simulink model "COSTEP"  (R2024b)
settings: Solver=FixedStepAuto  StartTime=0.0  StopTime=25  FixedStep=1/3600  RelTol=1e-3
model workspace (MAT data in the model file):
  AD : Simulink.Parameter (value not decoded)
  AG : Simulink.Parameter (value not decoded)
  AH : Simulink.Parameter (value not decoded)
  AV : Simulink.Parameter (value not decoded)
  AVP : Simulink.Parameter (value not decoded)
  BCHL : Simulink.Parameter (value not decoded)
  BCHV : Simulink.Parameter (value not decoded)
  BD : Simulink.Parameter (value not decoded)
  BDIST : Simulink.Parameter (value not decoded)
  BG : Simulink.Parameter (value not decoded)
  BH : Simulink.Parameter (value not decoded)
  BVP : Simulink.Parameter (value not decoded)
  CD : Simulink.Parameter (value not decoded)
  CDIST : Simulink.Parameter (value not decoded)
  CG : Simulink.Parameter (value not decoded)
  CH : Simulink.Parameter (value not decoded)
  CVP : Simulink.Parameter (value not decoded)
  DDIST : Simulink.Parameter (value not decoded)
  DIST_CONST : Simulink.Parameter (value not decoded)
  ISV : Simulink.Parameter (value not decoded)
  TLAST : Simulink.Parameter (value not decoded)
  TNEXT : Simulink.Parameter (value not decoded)
  XMW : Simulink.Parameter (value not decoded)
  XNS : Simulink.Parameter (value not decoded)
  XNS2 : Simulink.Parameter (value not decoded)
  XNS3 : Simulink.Parameter (value not decoded)
  XNSADD : Simulink.Parameter (value not decoded)
  XNSE : Simulink.Parameter (value not decoded)
symbols that are objects in the model workspace (value not decoded): AD, AG, AH, AV, AVP, BD, BG, BH, BVP, CD, CG, CH, CVP, XMW, XNS, XNS2, XNS3, XNSE
undefined symbols (not defined in the file or in its folder): magnitude, msgbox, SETPT, XMEAS, XMV
libraries: mylib x381, dspindex x31
(part 4 of 12)

== system COSTEP/Stripper/PTC Pressure of Liquid zone in stripper mmHg ==
  XLC : Inport
  TCC : Inport  Port=2
  Bus Creator1 : BusCreator  Inputs=8
  Demux : Demux  Outputs=8
  PPR(I) : Product
  PTR Total Pressure of Reactor mmHg : Sum  Inputs=+
  VPR Vapour Pressure mmHg : Subsystem
  PTC : Outport  PortDimensions=1  VectorParamsAs1DForOutWhenUnconnected=off
  wires:
  Demux/1 -> Bus Creator1/1  "PPR(1)"
  Demux/2 -> Bus Creator1/2  "PPR(2)"
  Demux/7 -> Bus Creator1/7  "PPR(7)"
  TCC/1 -> VPR Vapour Pressure mmHg/1(TCR)
  Demux/8 -> Bus Creator1/8  "PPR(8)"
  PPR(I)/1 -> Demux/1
  VPR Vapour Pressure mmHg/1(VPR) -> PPR(I)/2
  PTR Total Pressure of Reactor mmHg/1 -> PTC/1
  XLC/1 -> PPR(I)/1
  Bus Creator1/1 -> PTR Total Pressure of Reactor mmHg/1
  Demux/6 -> Bus Creator1/6  "PPR(6)"
  Demux/4 -> Bus Creator1/4  "PPR(4)"
  Demux/5 -> Bus Creator1/5  "PPR(5)"
  Demux/3 -> Bus Creator1/3  "PPR(3)"

== system COSTEP/Stripper/Position of Valve 8 % ==
  Bus Selector : BusSelector  OutputSignals=XMV(8)
  Bus Selector1 : BusSelector  OutputSignals=IDV(19)
  Constant : Constant  Value=46
  Control valve : mylib/Control valve  SystemSampleTime=-1  VariantActivationTime=update diagram  AllowFlexibleInterface=on  Latency=0  AutoFrameSizeCalculation=off
  Divide : Product  Inputs=*/
  Initial state variable : mylib/Initial state variable
  Integration : mylib/Integration  SystemSampleTime=-1  VariantActivationTime=update diagram  AllowFlexibleInterface=on  Latency=0  AutoFrameSizeCalculation=off
  Subtract : Sum  Inputs=+-
  VTAU(8) : Constant  Value=5/3600
  "YY(46) " : Outport  PortDimensions=1  VectorParamsAs1DForOutWhenUnconnected=off
  wires:
  Integration/1 -> "YY(46) "/1, Subtract/2  "VPOS(8)"
  Subtract/1 -> Divide/1
  Control valve/1 -> Subtract/1
  VTAU(8)/1 -> Divide/2
  Divide/1 -> Integration/1
  Initial state variable/1 -> Integration/2
  [XMV] -> Bus Selector/1
  Bus Selector/1 -> Control valve/1  "<XMV(8)>"
  [IDV] -> Bus Selector1/1
  Bus Selector1/1 -> Control valve/2  "<IDV(19)>"
  Constant/1 -> Initial state variable/1

== system COSTEP/Stripper/Position of Valve 9 % ==
  Bus Selector : BusSelector  OutputSignals=XMV(9)
  Bus Selector1 : BusSelector  OutputSignals=IDV(19)
  Constant : Constant  Value=47
  Control valve : mylib/Control valve  SystemSampleTime=-1  VariantActivationTime=update diagram  AllowFlexibleInterface=on  Latency=0  AutoFrameSizeCalculation=off
  Divide : Product  Inputs=*/
  Initial state variable : mylib/Initial state variable
  Integration : mylib/Integration  SystemSampleTime=-1  VariantActivationTime=update diagram  AllowFlexibleInterface=on  Latency=0  AutoFrameSizeCalculation=off
  Subtract : Sum  Inputs=+-
  VTAU(9) : Constant  Value=120/3600
  "YY(47) " : Outport  PortDimensions=1  VectorParamsAs1DForOutWhenUnconnected=off
  wires:
  Integration/1 -> "YY(47) "/1, Subtract/2  "VPOS(9)"
  Subtract/1 -> Divide/1
  Control valve/1 -> Subtract/1
  VTAU(9)/1 -> Divide/2
  Divide/1 -> Integration/1
  Initial state variable/1 -> Integration/2
  [XMV] -> Bus Selector/1
  Bus Selector/1 -> Control valve/1  "<XMV(9)>"
  Bus Selector1/1 -> Control valve/2  "<IDV(19)>"
  [IDV] -> Bus Selector1/1
  Constant/1 -> Initial state variable/1

== system COSTEP/Stripper/Split Fractions ==
  Bus Creator1 : BusCreator  Inputs=4
  SFR(1) : Constant  Value=0.99500
  SFR(2) : Constant  Value=0.99100
  SFR(3) : Constant  Value=0.99000
  Split fraction : Subsystem
  SFR : Outport  VectorParamsAs1DForOutWhenUnconnected=off
  wires:
  Bus Creator1/1 -> SFR/1
  SFR(2)/1 -> Bus Creator1/2
  Split fraction/1(SFR) -> Bus Creator1/4
  SFR(1)/1 -> Bus Creator1/1
  SFR(3)/1 -> Bus Creator1/3

== system COSTEP/Stripper/Stream 12 ==
  FCM(I,12) : Inport
  Bus Creator : BusCreator  Inputs=5
  Display : Display
  FTM(12) : Sum  Inputs=+
  Gain : Gain
  HST(12) Molar Enthalpy of Stream 12 MBtu/lb-mol : Subsystem
  ITY : Constant  Value=0
  XST(I,12) : Product  Inputs=*/
  wires:
  FTM(12)/1 -> XST(I,12)/2, Bus Creator/4  "FTM(12)"
  FCM(I,12)/1 -> XST(I,12)/1, Bus Creator/5, FTM(12)/1  "FCM(I;12)"
  XST(I,12)/1 -> Bus Creator/1, HST(12) Molar Enthalpy of Stream 12 MBtu/lb-mol/3(XST(I,I))  "XST(I;12)"
  [TCC] -> Gain/1
  Gain/1 -> Bus Creator/2, HST(12) Molar Enthalpy of Stream 12 MBtu/lb-mol/2(T)  "TST(12)"
  ITY/1 -> HST(12) Molar Enthalpy of Stream 12 MBtu/lb-mol/1(ITY)
  HST(12) Molar Enthalpy of Stream 12 MBtu/lb-mol/1("H ") -> Bus Creator/3  "HST(12)"
  Bus Creator/1 -> Display/1

== system COSTEP/Stripper/Stream 13 ==
  XST(I,13) : Inport  PortDimensions=8
  TST(13) : Inport  Port=2
  VPOS(8) : Inport  Port=3
  PTC : Inport  Port=4
  "   " : Constant  Value=100
  Bus Creator : BusCreator  Inputs=7
  FCM(I,13) Component molar flow of Stream 13 lb-mol/h : Product
  FTM(13) : Product  Inputs=**/
  HST(13) Molar Enthalpy of Stream 13 MBtu/lb-mol : Subsystem
  ITY : Constant  Value=0
  VRNG(8) : Constant  Value=1000
  Properties of Stream 13 : Outport  VectorParamsAs1DForOutWhenUnconnected=off
  wires:
  FTM(13)/1 -> Bus Creator/4, FCM(I,13) Component molar flow of Stream 13 lb-mol/h/2  "FTM(13)"
  ITY/1 -> Bus Creator/6, HST(13) Molar Enthalpy of Stream 13 MBtu/lb-mol/1(ITY)  "Phase"
  XST(I,13)/1 -> Bus Creator/1, FCM(I,13) Component molar flow of Stream 13 lb-mol/h/1, HST(13) Molar Enthalpy of Stream 13 MBtu/lb-mol/3(XST(I,I))  "XST(I;13)"
  HST(13) Molar Enthalpy of Stream 13 MBtu/lb-mol/1("H ") -> Bus Creator/3  "HST(13)"
  TST(13)/1 -> Bus Creator/2, HST(13) Molar Enthalpy of Stream 13 MBtu/lb-mol/2(T)  "TST(13)"
  VPOS(8)/1 -> FTM(13)/1
  FCM(I,13) Component molar flow of Stream 13 lb-mol/h/1 -> Bus Creator/5  "FCM(I;13)"
  VRNG(8)/1 -> FTM(13)/2
  "   "/1 -> FTM(13)/3
  Bus Creator/1 -> Properties of Stream 13/1
  PTC/1 -> Bus Creator/7  "PTC"

== system COSTEP/Stripper/Stream 5 ==
  FCM(I,5) : Inport
  Bus Creator : BusCreator  Inputs=7
  FTM(5) : Sum  Inputs=+
  HST(5) Molar Enthalpy of Stream 5 MBtu/lb-mol : Subsystem
  ITY : Constant
  XST(I,5) : Product  Inputs=*/
  Properties of Stream 5 : Outport  VectorParamsAs1DForOutWhenUnconnected=off
  tag scope: PropertiesStream5=global
  wires:
  FTM(5)/1 -> Bus Creator/4, XST(I,5)/2  "FTM(5)"
  FCM(I,5)/1 -> XST(I,5)/1, Bus Creator/5, FTM(5)/1  "FCM(I;5)"
  XST(I,5)/1 -> Bus Creator/1, HST(5) Molar Enthalpy of Stream 5 MBtu/lb-mol/3(XST(I,5))  "XST(I;5)"
  [TCC] -> Bus Creator/2, HST(5) Molar Enthalpy of Stream 5 MBtu/lb-mol/2(TST(5))  "TST(5)"
  ITY/1 -> Bus Creator/6, HST(5) Molar Enthalpy of Stream 5 MBtu/lb-mol/1(ITY)  "Phase"
  HST(5) Molar Enthalpy of Stream 5 MBtu/lb-mol/1("H ") -> Bus Creator/3  "HST(5)"
  Bus Creator/1 -> [PropertiesStream5], Properties of Stream 5/1
  [PTV] -> Bus Creator/7

== system COSTEP/Stripper/TCC Initial Temperature in Stripper °C  ==
  UTLC : Inport  PortDimensions=1
  ETC : Inport  Port=2  PortDimensions=1
  XLC : Inport  Port=3  PortDimensions=8
  "AG(I) Coefficient A to determine Enthalpy MBtu/lb·°F " : Constant  Value=[3.411e-6;0.3799e-6;0.2491e-6;0.3567e-6;0.3463e-6;0.393e-6;0.17e-6;0.15e-6]
  "AH(I) Coefficient A to determine Enthalpy MBtu/lb·°F " : Constant  Value=[1e-6;1e-6;1e-6;0.96e-6;0.573e-6;0.652e-6;0.515e-6;0.471e-6]
  AV(I) Coefficient AV to determine Enthalpy MBtu/lb : Constant  Value=[1e-6;1e-6;1e-6;86.7e-6;160e-6;160e-6;225e-6;209e-6]
  BG(I) Coefficient B to determine Enthalpy MBtu/lb·°F² : Constant  Value=[7.18e-10;1.08e-9;1.36e-11;8.51e-10;8.96e-10;1.02e-9;0;0]
  BH(I) Coefficient B to determine Enthalpy MBtu/lb·°F² : Constant  Value=[0;0;0;8.7e-9;2.41e-9;2.18e-9;5.65e-10;8.7e-10]
  CG(I) Coefficient C to determine Enthalpy MBtu/lb·°F³ : Constant  Value=[6e-13;-3.98e-13;-3.93e-14;-3.12e-13;-3.27e-13;-3.12e-13;0;0]
  CH(I) Coefficient C to determine Enthalpy MBtu/lb·°F³ : Constant  Value=[0;0;0;4.81e-11;1.82e-11;1.94e-11;3.82e-12;2.62e-12]
  Delay : Delay  DelayLength=1  InitialCondition=0
  ITY : Constant  Value=0
  MATLAB Function : MATLAB Function  TreatAsAtomicUnit=on
  "XMW(I) Molecular weight of components lb/lb-mol " : Constant  Value=[2;25.4;28;32;46;48;62;76]
  TCC : Outport  PortDimensions=1  VectorParamsAs1DForOutWhenUnconnected=off
  wires:
  MATLAB Function/1(TCC) -> Delay/1, TCC/1
  Delay/1 -> MATLAB Function/13("TCC ")
  "AG(I) Coefficient A to determine Enthalpy MBtu/lb·°F "/1 -> MATLAB Function/4(AG)
  AV(I) Coefficient AV to determine Enthalpy MBtu/lb/1 -> MATLAB Function/7(AV)
  ETC/1 -> MATLAB Function/10(ETC)
  CH(I) Coefficient C to determine Enthalpy MBtu/lb·°F³/1 -> MATLAB Function/3(CH)
  UTLC/1 -> MATLAB Function/11(UTLC)
  ITY/1 -> MATLAB Function/12(ITY)
  "XMW(I) Molecular weight of components lb/lb-mol "/1 -> MATLAB Function/8(XMW)
  XLC/1 -> MATLAB Function/9(XLC)
  "AH(I) Coefficient A to determine Enthalpy MBtu/lb·°F "/1 -> MATLAB Function/1(AH)
  CG(I) Coefficient C to determine Enthalpy MBtu/lb·°F³/1 -> MATLAB Function/6(CG)
  BH(I) Coefficient B to determine Enthalpy MBtu/lb·°F²/1 -> MATLAB Function/2(BH)
  BG(I) Coefficient B to determine Enthalpy MBtu/lb·°F²/1 -> MATLAB Function/5(BG)

== system COSTEP/Stripper/Volume of Stripper ==
  UTLC : Inport  PortDimensions=1
  XLC : Inport  Port=2  PortDimensions=8
  "DLC Molar Density of Liquids in Stripper lb-mol/ft³    " : Subsystem
  "VLC Liquid Volume in Stripper ft³ " : Product  Inputs=*/
  tag scope: DLC=global, VLC=global
  wires:
  "DLC Molar Density of Liquids in Stripper lb-mol/ft³    "/1("DLC ") -> [DLC], "VLC Liquid Volume in Stripper ft³ "/2
  XLC/1 -> "DLC Molar Density of Liquids in Stripper lb-mol/ft³    "/1(XLC)
  "VLC Liquid Volume in Stripper ft³ "/1 -> [VLC]
  [TCC] -> "DLC Molar Density of Liquids in Stripper lb-mol/ft³    "/2(TCC)
  UTLC/1 -> "VLC Liquid Volume in Stripper ft³ "/1

== system COSTEP/Valve/FTM(1) Total molar flow of Stream 1 lb-mol//h ==
  VPOS(1) : Inport
  VRNG(1) : Inport  Port=2
  " " : Product  Inputs=**/
  Constant : Constant  Value=100
  FTM(1) : Outport  PortDimensions=1  VectorParamsAs1DForOutWhenUnconnected=off
  wires:
  VRNG(1)/1 -> " "/2
  Constant/1 -> " "/3
  VPOS(1)/1 -> " "/1
  " "/1 -> FTM(1)/1

== system COSTEP/Valve/Position of Valve 1 % ==
  Bus Selector : BusSelector  OutputSignals=XMV(1)
  Constant : Constant  Value=39
  Control valve : mylib/Control valve  SystemSampleTime=-1  VariantActivationTime=update diagram  AllowFlexibleInterface=on  Latency=0  AutoFrameSizeCalculation=off
  Divide : Product  Inputs=*/
  IVST(1) : Constant  Value=0
  Initial state variable : mylib/Initial state variable
  Integration : mylib/Integration  SystemSampleTime=-1  VariantActivationTime=update diagram  AllowFlexibleInterface=on  Latency=0  AutoFrameSizeCalculation=off
  Subtract : Sum  Inputs=+-
  VTAU(1) : Constant  Value=8/3600
  "YY(39) " : Outport  VectorParamsAs1DForOutWhenUnconnected=off
  wires:
  Integration/1 -> "YY(39) "/1, Subtract/2  "VPOS(1)"
  Subtract/1 -> Divide/1
  VTAU(1)/1 -> Divide/2
  Divide/1 -> Integration/1
  Control valve/1 -> Subtract/1
  [XMV] -> Bus Selector/1
  Bus Selector/1 -> Control valve/1  "<XMV(1)>"
  IVST(1)/1 -> Control valve/2
  Constant/1 -> Initial state variable/1
  Initial state variable/1 -> Integration/2

== system COSTEP/Valve 2/FTM(2) Total molar flow of Stream 2 lb-mol//h ==
  VPOS(2) : Inport
  VRNG(2) : Inport  Port=2
  " " : Product  Inputs=**/
  Constant : Constant  Value=100
  FTM(2) : Outport  PortDimensions=1  VectorParamsAs1DForOutWhenUnconnected=off
  wires:
  VRNG(2)/1 -> " "/2
  Constant/1 -> " "/3
  VPOS(2)/1 -> " "/1
  " "/1 -> FTM(2)/1

== system COSTEP/Valve 2/Position of Valve 2 % ==
  Bus Selector : BusSelector  OutputSignals=XMV(2)
  Constant : Constant  Value=40
  Control valve : mylib/Control valve  SystemSampleTime=-1  VariantActivationTime=update diagram  AllowFlexibleInterface=on  Latency=0  AutoFrameSizeCalculation=off
  Divide : Product  Inputs=*/
  IVST(2) : Constant  Value=0
  Initial state variable : mylib/Initial state variable
  Integration : mylib/Integration  SystemSampleTime=-1  VariantActivationTime=update diagram  AllowFlexibleInterface=on  Latency=0  AutoFrameSizeCalculation=off
  Subtract : Sum  Inputs=+-
  VTAU(2) : Constant  Value=8/3600
  "YY(40)  " : Outport  VectorParamsAs1DForOutWhenUnconnected=off
  wires:
  Control valve/1 -> Subtract/1
  Subtract/1 -> Divide/1
  VTAU(2)/1 -> Divide/2
  Divide/1 -> Integration/1
  Integration/1 -> Subtract/2, "YY(40)  "/1  "VPOS(2)"
  Initial state variable/1 -> Integration/2
  [XMV] -> Bus Selector/1
  Bus Selector/1 -> Control valve/1  "<XMV(2)>"
  IVST(2)/1 -> Control valve/2
  Constant/1 -> Initial state variable/1

== system COSTEP/Valve 3/FTM(3) Total molar flow of Stream 3 lb-mol//h ==
  VPOS(3) : Inport
  VRNG(3) : Inport  Port=2
  " " : Product  Inputs=***/
  Bus Selector : BusSelector  OutputSignals=IDV(6)
  Constant : Constant  Value=100
  Constant1 : Constant
  Subtract : Sum  Inputs=+-
  FTM(3) : Outport  PortDimensions=1  VectorParamsAs1DForOutWhenUnconnected=off
  wires:
  VPOS(3)/1 -> " "/1
  " "/1 -> FTM(3)/1
  Constant1/1 -> Subtract/1
  [IDV] -> Bus Selector/1
  Constant/1 -> " "/4
  Subtract/1 -> " "/2
  VRNG(3)/1 -> " "/3
  Bus Selector/1 -> Subtract/2  "<IDV(6)>"

== system COSTEP/Valve 3/Position of Valve 3 % ==
  Bus Selector : BusSelector  OutputSignals=XMV(3)
  Constant : Constant  Value=41
  Control valve : mylib/Control valve  SystemSampleTime=-1  VariantActivationTime=update diagram  AllowFlexibleInterface=on  Latency=0  AutoFrameSizeCalculation=off
  Divide : Product  Inputs=*/
  IVST(3) : Constant  Value=0
  Initial state variable : mylib/Initial state variable
  Integration : mylib/Integration  SystemSampleTime=-1  VariantActivationTime=update diagram  AllowFlexibleInterface=on  Latency=0  AutoFrameSizeCalculation=off
  Subtract : Sum  Inputs=+-
  VTAU(3) : Constant  Value=6/3600
  "YY(41) " : Outport  VectorParamsAs1DForOutWhenUnconnected=off
  wires:
  Control valve/1 -> Subtract/1
  Subtract/1 -> Divide/1
  VTAU(3)/1 -> Divide/2
  Divide/1 -> Integration/1
  Integration/1 -> "YY(41) "/1, Subtract/2  "VPOS(3)"
  Initial state variable/1 -> Integration/2
  [XMV] -> Bus Selector/1
  Bus Selector/1 -> Control valve/1  "<XMV(3)>"
  IVST(3)/1 -> Control valve/2
  Constant/1 -> Initial state variable/1

== system COSTEP/Valve 4/FTM(4) Total molar flow of Stream 4 lb-mol//h ==
  VPOS(4) : Inport
  VRNG(4) : Inport  Port=2
  " " : Product  Inputs=***/
  Add : Sum
  Bus Selector : BusSelector  OutputSignals=IDV(7)
  Constant : Constant
  Constant1 : Constant  Value=0.2
  Constant3 : Constant  Value=100
  Constant4 : Constant  Value=1e-10
  Product1 : Product
  Subtract : Sum  Inputs=+-
  FTM(4) : Outport  PortDimensions=1  VectorParamsAs1DForOutWhenUnconnected=off
  wires:
  Add/1 -> FTM(4)/1
  Constant4/1 -> Add/2
  " "/1 -> Add/1
  VPOS(4)/1 -> " "/1
  Bus Selector/1 -> Product1/1  "<IDV(7)>"
  Product1/1 -> Subtract/2
  Constant1/1 -> Product1/2
  Constant/1 -> Subtract/1
  Constant3/1 -> " "/4
  VRNG(4)/1 -> " "/3
  Subtract/1 -> " "/2
  [IDV] -> Bus Selector/1

== system COSTEP/Valve 4/Position of Valve 4 % ==
  Bus Selector : BusSelector  OutputSignals=XMV(4)
  Constant : Constant  Value=42
  Control valve : mylib/Control valve  SystemSampleTime=-1  VariantActivationTime=update diagram  AllowFlexibleInterface=on  Latency=0  AutoFrameSizeCalculation=off
  Divide : Product  Inputs=*/
  IVST(4) : Constant  Value=0
  Initial state variable : mylib/Initial state variable
  Integration : mylib/Integration  SystemSampleTime=-1  VariantActivationTime=update diagram  AllowFlexibleInterface=on  Latency=0  AutoFrameSizeCalculation=off
  Subtract : Sum  Inputs=+-
  VTAU(4) : Constant  Value=9/3600
  "YY(42) " : Outport  VectorParamsAs1DForOutWhenUnconnected=off
  wires:
  Control valve/1 -> Subtract/1
  Subtract/1 -> Divide/1
  VTAU(4)/1 -> Divide/2
  Divide/1 -> Integration/1
  Integration/1 -> "YY(42) "/1, Subtract/2  "VPOS(4)"
  Initial state variable/1 -> Integration/2
  [XMV] -> Bus Selector/1
  Bus Selector/1 -> Control valve/1  "<XMV(4)>"
  IVST(4)/1 -> Control valve/2
  Constant/1 -> Initial state variable/1

== system COSTEP/Compressor/Subsystem/If Action Subsystem ==
  In1 : Inport
  Action Port : ActionPort  ActionPortLabel=if(u1 < 1)
  Out1 : Outport  VectorParamsAs1DForOutWhenUnconnected=off
  wires:
  In1/1 -> Out1/1

== system COSTEP/Compressor/Subsystem/If Action Subsystem1 ==
  In1 : Inport
  Action Port : ActionPort  ActionPortLabel=elseif(u1>1.3)
  Out1 : Outport  VectorParamsAs1DForOutWhenUnconnected=off
  wires:
  In1/1 -> Out1/1

== system COSTEP/Compressor/Subsystem/If Action Subsystem2 ==
  In1 : Inport
  Action Port : ActionPort  ActionPortLabel=else
  Out1 : Outport  VectorParamsAs1DForOutWhenUnconnected=off
  wires:
  In1/1 -> Out1/1

== system COSTEP/Condenser/Cooling water outlet temperature/TCWS Inlet temperature of cooling water °C ==
  Add : Sum
  Bus Selector : BusSelector  OutputSignals=signal1.TESUB8(6)
  Bus Selector1 : BusSelector  OutputSignals=IDV(5)
  Constant : Constant  Value=5
  Product1 : Product
  TCWS : Outport  VectorParamsAs1DForOutWhenUnconnected=off
  wires:
  Constant/1 -> Product1/2
  Bus Selector/1 -> Add/1  "<TESUB8(6)>"
  Bus Selector1/1 -> Product1/1  "<IDV(5)>"
  [TESUB8] -> Bus Selector/1
  Product1/1 -> Add/2
  [IDV] -> Bus Selector1/1
  Add/1 -> TCWS/1

== system COSTEP/Control Mode/Braatz/  ==
  XMEAS : Inport
  Bus Selector : BusSelector  OutputSignals=signal1.XMEAS(2),signal8.XMEAS(26)
  CONTROL 1 : Subsystem  Priority=1
  CONTROL 14 : Subsystem  Priority=2
  XMV(1) : Outport  VectorParamsAs1DForOutWhenUnconnected=off
  wires:
  CONTROL 1/1(XMV(1)) -> XMV(1)/1
  XMEAS/1 -> Bus Selector/1
  Bus Selector/1 -> CONTROL 1/1(XMEAS(2))  "<XMEAS(2)>"
  Bus Selector/2 -> CONTROL 14/1(XMEAS(26))  "<XMEAS(26)>"
  CONTROL 14/1(SETPT(1)) -> CONTROL 1/2(SETPT(1))

== system COSTEP/Control Mode/Braatz/ 1 ==
  XMEAS : Inport
  Bus Selector : BusSelector  OutputSignals=signal1.XMEAS(3),signal8.XMEAS(27)
  CONTROL 15 : Subsystem
  CONTROL 2 : Subsystem
  XMV(2) : Outport  VectorParamsAs1DForOutWhenUnconnected=off
  wires:
  CONTROL 2/1(XMV(2)) -> XMV(2)/1
  XMEAS/1 -> Bus Selector/1
  Bus Selector/1 -> CONTROL 2/1(XMEAS(2))  "<XMEAS(3)>"
  Bus Selector/2 -> CONTROL 15/1(XMEAS(27))  "<XMEAS(27)>"
  CONTROL 15/1(SETPT(2)) -> CONTROL 2/2(SETPT(2))

== system COSTEP/Control Mode/Braatz/ 10 ==
  XMEAS : Inport
  Bus Selector : BusSelector  OutputSignals=signal9.XMEAS(30)
  CONTROL 19 : Subsystem
  CONTROL 6 : Subsystem
  XMV(6) : Outport  VectorParamsAs1DForOutWhenUnconnected=off
  wires:
  CONTROL 6/1(XMV(6)) -> XMV(6)/1
  XMEAS/1 -> CONTROL 6/2(XMEAS), Bus Selector/1
  Bus Selector/1 -> CONTROL 19/1(XMEAS(30))  "<XMEAS(30)>"
  CONTROL 19/1(SETPT(6)) -> CONTROL 6/1(SETPT(6))

== system COSTEP/Control Mode/Braatz/ 2 ==
  XMEAS : Inport
  Bus Selector : BusSelector  OutputSignals=signal1.XMEAS(1),signal8.XMEAS(23)
  CONTROL 13 : Subsystem
  CONTROL 3 : Subsystem
  XMV(3) : Outport  VectorParamsAs1DForOutWhenUnconnected=off
  wires:
  CONTROL 3/1(XMV(3)) -> XMV(3)/1
  XMEAS/1 -> Bus Selector/1
  Bus Selector/1 -> CONTROL 3/1(XMEAS(1))  "<XMEAS(1)>"
  Bus Selector/2 -> CONTROL 13/1(XMEAS(23))  "<XMEAS(23)>"
  CONTROL 13/1(SETPT(3)) -> CONTROL 3/2(SETPT(3))

== system COSTEP/Control Mode/Braatz/ 3 ==
  XMEAS : Inport
  Bus Selector : BusSelector  OutputSignals=signal1.XMEAS(4),signal2.XMEAS(8)
  CONTROL 17 : Subsystem
  CONTROL 4 : Subsystem
  XMV(4) : Outport  VectorParamsAs1DForOutWhenUnconnected=off
  wires:
  CONTROL 4/1(XMV(4)) -> XMV(4)/1
  XMEAS/1 -> Bus Selector/1
  Bus Selector/1 -> CONTROL 4/1(XMEAS(4))  "<XMEAS(4)>"
  Bus Selector/2 -> CONTROL 17/1(XMEAS(8))  "<XMEAS(8)>"
  CONTROL 17/1(SETPT(4)) -> CONTROL 4/2(SETPT(4))

== system COSTEP/Control Mode/Braatz/ 4 ==
  XMEAS : Inport
  Bus Selector : BusSelector  OutputSignals=signal1.XMEAS(5)
  CONTROL 5 : Subsystem
  XMV(5) : Outport  VectorParamsAs1DForOutWhenUnconnected=off
  wires:
  CONTROL 5/1(XMV(5)) -> XMV(5)/1
  XMEAS/1 -> Bus Selector/1
  Bus Selector/1 -> CONTROL 5/1(XMEAS(5))  "<XMEAS(5)>"

== system COSTEP/Control Mode/Braatz/ 5 ==
  XMEAS : Inport
  Bus Selector : BusSelector  OutputSignals=signal3.XMEAS(12)
  CONTROL 7 : Subsystem
  XMV(7) : Outport  VectorParamsAs1DForOutWhenUnconnected=off
  wires:
  CONTROL 7/1(XMV(7)) -> XMV(7)/1
  XMEAS/1 -> Bus Selector/1
  Bus Selector/1 -> CONTROL 7/1(XMEAS(12))  "<XMEAS(12)>"

== system COSTEP/Control Mode/Braatz/ 6 ==
  XMEAS : Inport
  Bus Selector : BusSelector  OutputSignals=signal4.XMEAS(15)
  CONTROL 8 : Subsystem
  XMV(8) : Outport  VectorParamsAs1DForOutWhenUnconnected=off
  wires:
  CONTROL 8/1(XMV(8)) -> XMV(8)/1
  XMEAS/1 -> Bus Selector/1
  Bus Selector/1 -> CONTROL 8/1(XMEAS(15))  "<XMEAS(15)>"

== system COSTEP/Control Mode/Braatz/ 7 ==
  XMEAS : Inport
  Bus Selector : BusSelector  OutputSignals=signal4.XMEAS(17)
  CONTROL 11 : Subsystem
  XMV(11) : Outport  VectorParamsAs1DForOutWhenUnconnected=off
  wires:
  CONTROL 11/1(XMV(11)) -> XMV(11)/1
  XMEAS/1 -> Bus Selector/1
  Bus Selector/1 -> CONTROL 11/1(XMEAS(17))  "<XMEAS(17)>"

== system COSTEP/Control Mode/Braatz/ 8 ==
  XMEAS : Inport
  Bus Selector : BusSelector  OutputSignals=XMEAS(21),signal2.XMEAS(9)
  CONTROL 10 : Subsystem
  CONTROL 18 : Subsystem
  XMV(10) : Outport  VectorParamsAs1DForOutWhenUnconnected=off
  wires:
  CONTROL 10/1(XMV(10)) -> XMV(10)/1
  XMEAS/1 -> Bus Selector/1
  Bus Selector/1 -> CONTROL 10/1(XMEAS(21))  "<XMEAS(21)>"
  Bus Selector/2 -> CONTROL 18/1(XMEAS(9))  "<XMEAS(9)>"
  CONTROL 18/1(SETPT(10)) -> CONTROL 10/2(SETPT(10))

== system COSTEP/Control Mode/Braatz/ 9 ==
  XMEAS : Inport
  Bus Selector : BusSelector  OutputSignals=signal4.XMEAS(19),signal4.XMEAS(18),signal10.XMEAS(38)
  CONTROL 16 : Subsystem
  CONTROL 20 : Subsystem
  CONTROL 9 : Subsystem
  XMV(9) : Outport  VectorParamsAs1DForOutWhenUnconnected=off
  wires:
  CONTROL 9/1(XMV(9)) -> XMV(9)/1
  XMEAS/1 -> Bus Selector/1
  Bus Selector/1 -> CONTROL 9/1(XMEAS(19))  "<XMEAS(19)>"
  Bus Selector/2 -> CONTROL 16/1(XMEAS(18))  "<XMEAS(18)>"
  Bus Selector/3 -> CONTROL 20/1(XMEAS(38))  "<XMEAS(38)>"
  CONTROL 16/1(SETPT(9)) -> CONTROL 9/2(SETPT(9))
  CONTROL 20/1(SETPT(16)) -> CONTROL 16/2(SETPT(16))

== system COSTEP/Mixing Zone/Holdup of Components in Mixing Zone/Holdup of Vapour Components in the Mixing Zone ==
  note: UCVV(8)
      | Holdup of Component H (Vapour) in Mixing zone
      | lb-mol
  note: UCVV(7)
      | Holdup of Component G (Vapour) in Mixing zone
      | lb-mol
  note: UCVV(6)
      | Holdup of Component F (Vapour) in Mixing zone
      | lb-mol
  note: UCVV(5)
      | Holdup of Component E (Vapour) in Mixing zone
      | lb-mol
  note: UCVV(4)
      | Holdup of Component D (Vapour) in Mixing zone
      | lb-mol
  note: UCVV(3)
      | Holdup of Component C (Vapour) in Mixing zone
      | lb-mol
  note: UCVV(2)
      | Holdup of Component B (Vapour) in Mixing zone
      | lb-mol
  note: UCVV(1)
      | Holdup of Component A (Vapour) in Mixing zone
      | lb-mol
  YY(28:35) : Inport
  Bus Creator : BusCreator  Inputs=8
  Bus Selector4 : BusSelector  OutputSignals=YY(28),YY(29),YY(30),YY(31),YY(32),YY(33),YY(34),YY(35)
  UCVV : Outport  VectorParamsAs1DForOutWhenUnconnected=off
  wires:
  Bus Selector4/7 -> Bus Creator/7  "<YY(34)>"
  Bus Selector4/2 -> Bus Creator/2  "<YY(29)>"
  Bus Selector4/3 -> Bus Creator/3  "<YY(30)>"
  Bus Selector4/4 -> Bus Creator/4  "<YY(31)>"
  Bus Selector4/5 -> Bus Creator/5  "<YY(32)>"
  Bus Selector4/6 -> Bus Creator/6  "<YY(33)>"
  Bus Selector4/1 -> Bus Creator/1  "<YY(28)>"
  Bus Selector4/8 -> Bus Creator/8  "<YY(35)>"
  YY(28:35)/1 -> Bus Selector4/1
  Bus Creator/1 -> UCVV/1

== system COSTEP/Mixing Zone/Holdup of Components in Mixing Zone/Subsystem ==
  Properties of Stream 1 : Inport
  Bus Creator : BusCreator  Inputs=8
  Bus Selector : BusSelector  OutputSignals=FCM(I;1)
  Multiport Selector : dspindex/Multiport Selector  rowsOrCols=Rows  idxCellArray={ 1,2,3,4,5,6,7,8}  idxErrMode=Clip Index
  FCM(I;1) : Outport  VectorParamsAs1DForOutWhenUnconnected=off
  wires:
  Multiport Selector/1 -> Bus Creator/1  "FCM(1;1)"
  Multiport Selector/2 -> Bus Creator/2  "FCM(2;1)"
  Multiport Selector/8 -> Bus Creator/8  "FCM(8;1)"
  Multiport Selector/6 -> Bus Creator/6  "FCM(6;1)"
  Multiport Selector/7 -> Bus Creator/7  "FCM(7;1)"
  Multiport Selector/4 -> Bus Creator/4  "FCM(4;1)"
  Multiport Selector/5 -> Bus Creator/5  "FCM(5;1)"
  Multiport Selector/3 -> Bus Creator/3  "FCM(3;1)"
  Bus Selector/1 -> Multiport Selector/1  "<FCM(I;1)>"
  Properties of Stream 1/1 -> Bus Selector/1
  Bus Creator/1 -> FCM(I;1)/1

== system COSTEP/Mixing Zone/Holdup of Components in Mixing Zone/Subsystem1 ==
  Properties of Stream 2 : Inport
  Bus Creator : BusCreator  Inputs=8
  Bus Selector1 : BusSelector  OutputSignals=FCM(I;2)
  Multiport Selector1 : dspindex/Multiport Selector  rowsOrCols=Rows  idxCellArray={ 1,2,3,4,5,6,7,8}  idxErrMode=Clip Index
  FCM(I;2) : Outport  VectorParamsAs1DForOutWhenUnconnected=off
  wires:
  Multiport Selector1/5 -> Bus Creator/5  "FCM(5;2)"
  Bus Selector1/1 -> Multiport Selector1/1  "<FCM(I;2)>"
  Multiport Selector1/6 -> Bus Creator/6  "FCM(6;2)"
  Multiport Selector1/1 -> Bus Creator/1  "FCM(1;2)"
  Multiport Selector1/2 -> Bus Creator/2  "FCM(2;2)"
  Multiport Selector1/7 -> Bus Creator/7  "FCM(7;2)"
  Multiport Selector1/4 -> Bus Creator/4  "FCM(4;2)"
  Multiport Selector1/8 -> Bus Creator/8  "FCM(8;2)"
  Multiport Selector1/3 -> Bus Creator/3  "FCM(3;2)"
  Properties of Stream 2/1 -> Bus Selector1/1
  Bus Creator/1 -> FCM(I;2)/1

== system COSTEP/Mixing Zone/Holdup of Components in Mixing Zone/Subsystem2 ==
  Bus Creator : BusCreator  Inputs=8
  Bus Selector5 : BusSelector  OutputSignals=signal1.FCM(I;6) = FCM(I;7)
  Multiport Selector4 : dspindex/Multiport Selector  rowsOrCols=Rows  idxCellArray={ 1,2,3,4,5,6,7,8}  idxErrMode=Clip Index
  FCM(I;6) : Outport  VectorParamsAs1DForOutWhenUnconnected=off
  wires:
  Multiport Selector4/6 -> Bus Creator/6  "FCM(6;7)"
  Multiport Selector4/7 -> Bus Creator/7  "FCM(7;7)"
  Multiport Selector4/5 -> Bus Creator/5  "FCM(5;7)"
  Multiport Selector4/4 -> Bus Creator/4  "FCM(4;7)"
  Multiport Selector4/8 -> Bus Creator/8  "FCM(8;7)"
  Multiport Selector4/3 -> Bus Creator/3  "FCM(3;7)"
  Multiport Selector4/2 -> Bus Creator/2  "FCM(2;7)"
  [PropertiesStream6] -> Bus Selector5/1
  Multiport Selector4/1 -> Bus Creator/1  "FCM(1;7)"
  Bus Selector5/1 -> Multiport Selector4/1  "<FCM(I;6) = FCM(I;7)>"
  Bus Creator/1 -> FCM(I;6)/1

== system COSTEP/Mixing Zone/Holdup of Components in Mixing Zone/Subsystem3 ==
  Properties of Stream 3 : Inport
  Bus Creator : BusCreator  Inputs=8
  Bus Selector2 : BusSelector  OutputSignals=FCM(I;3)
  Multiport Selector2 : dspindex/Multiport Selector  rowsOrCols=Rows  idxCellArray={ 1,2,3,4,5,6,7,8}  idxErrMode=Clip Index
  FCM(I;3) : Outport  VectorParamsAs1DForOutWhenUnconnected=off
  wires:
  Multiport Selector2/2 -> Bus Creator/2  "FCM(2;3)"
  Multiport Selector2/4 -> Bus Creator/4  "FCM(4;3)"
  Multiport Selector2/8 -> Bus Creator/8  "FCM(8;3)"
  Bus Selector2/1 -> Multiport Selector2/1  "<FCM(I;3)>"
  Multiport Selector2/7 -> Bus Creator/7  "FCM(7;3)"
  Multiport Selector2/6 -> Bus Creator/6  "FCM(6;3)"
  Multiport Selector2/1 -> Bus Creator/1  "FCM(1;3)"
  Multiport Selector2/3 -> Bus Creator/3  "FCM(3;3)"
  Multiport Selector2/5 -> Bus Creator/5  "FCM(5;3)"
  Properties of Stream 3/1 -> Bus Selector2/1
  Bus Creator/1 -> FCM(I;3)/1

== system COSTEP/Mixing Zone/Holdup of Components in Mixing Zone/Subsystem4 ==
  Properties of Stream 5 : Inport
  Bus Creator : BusCreator  Inputs=8
  Bus Selector3 : BusSelector  OutputSignals=FCM(I;5)
  Multiport Selector3 : dspindex/Multiport Selector  rowsOrCols=Rows  idxCellArray={ 1,2,3,4,5,6,7,8}  idxErrMode=Clip Index
  FCM(I;5) : Outport  VectorParamsAs1DForOutWhenUnconnected=off
  wires:
  Multiport Selector3/6 -> Bus Creator/6  "FCM(6;5)"
  Multiport Selector3/8 -> Bus Creator/8  "FCM(8;5)"
  Multiport Selector3/5 -> Bus Creator/5  "FCM(5;5)"
  Multiport Selector3/2 -> Bus Creator/2  "FCM(2;5)"
  Bus Selector3/1 -> Multiport Selector3/1  "<FCM(I;5)>"
  Multiport Selector3/7 -> Bus Creator/7  "FCM(7;5)"
  Multiport Selector3/4 -> Bus Creator/4  "FCM(4;5)"
  Multiport Selector3/1 -> Bus Creator/1  "FCM(1;5)"
  Multiport Selector3/3 -> Bus Creator/3  "FCM(3;5)"
  Properties of Stream 5/1 -> Bus Selector3/1
  Bus Creator/1 -> FCM(I;5)/1

== system COSTEP/Mixing Zone/Holdup of Components in Mixing Zone/Subsystem5 ==
  Properties of Stream 9 : Inport
  Bus Creator : BusCreator  Inputs=8
  Bus Selector4 : BusSelector  OutputSignals=FCM(I;9)
  Multiport Selector5 : dspindex/Multiport Selector  rowsOrCols=Rows  idxCellArray={ 1,2,3,4,5,6,7,8}  idxErrMode=Clip Index
  FCM(I;9) : Outport  VectorParamsAs1DForOutWhenUnconnected=off
  wires:
  Multiport Selector5/7 -> Bus Creator/7  "FCM(7;9)"
  Multiport Selector5/6 -> Bus Creator/6  "FCM(6;9)"
  Multiport Selector5/8 -> Bus Creator/8  "FCM(8;9)"
  Bus Selector4/1 -> Multiport Selector5/1  "<FCM(I;9)>"
  Multiport Selector5/1 -> Bus Creator/1  "FCM(1;9)"
  Multiport Selector5/2 -> Bus Creator/2  "FCM(2;9)"
  Multiport Selector5/5 -> Bus Creator/5  "FCM(5;9)"
  Multiport Selector5/4 -> Bus Creator/4  "FCM(4;9)"
  Multiport Selector5/3 -> Bus Creator/3  "FCM(3;9)"
  Properties of Stream 9/1 -> Bus Selector4/1
  Bus Creator/1 -> FCM(I;9)/1

== system COSTEP/Mixing Zone/Holdup of Components in Mixing Zone/Vapour Holdup Fraction in the Mxing Zone ==
  UTVV : Inport
  UCVV : Inport  Port=2
  Bus Selector : BusSelector  OutputSignals=YY(28),YY(29),YY(30),YY(31),YY(32),YY(33),YY(34),YY(35)
  Mux : Mux  Inputs=8
  XVV(1) : Product  Inputs=*/
  XVV(2) : Product  Inputs=*/
  XVV(3) : Product  Inputs=*/
  XVV(4) : Product  Inputs=*/
  XVV(5) : Product  Inputs=*/
  XVV(6) : Product  Inputs=*/
  XVV(7) : Product  Inputs=*/
  XVV(8) : Product  Inputs=*/
  XVV : Outport  VectorParamsAs1DForOutWhenUnconnected=off
  wires:
  XVV(4)/1 -> Mux/4  "XVV(4)"
  UTVV/1 -> XVV(8)/2, XVV(7)/2, XVV(6)/2, XVV(5)/2, XVV(4)/2, XVV(3)/2, XVV(2)/2, XVV(1)/2
  XVV(8)/1 -> Mux/8  "XVV(8)"
  Bus Selector/3 -> XVV(3)/1  "<YY(30)>"
  XVV(5)/1 -> Mux/5  "XVV(5)"
  XVV(2)/1 -> Mux/2  "XVV(2)"
  XVV(7)/1 -> Mux/7  "XVV(7)"
  Bus Selector/8 -> XVV(8)/1  "<YY(35)>"
  XVV(6)/1 -> Mux/6  "XVV(6)"
  XVV(3)/1 -> Mux/3  "XVV(3)"
  Mux/1 -> XVV/1
  XVV(1)/1 -> Mux/1  "XVV(1)"
  Bus Selector/7 -> XVV(7)/1  "<YY(34)>"
  Bus Selector/5 -> XVV(5)/1  "<YY(32)>"
  Bus Selector/4 -> XVV(4)/1  "<YY(31)>"
  Bus Selector/2 -> XVV(2)/1  "<YY(29)>"
  Bus Selector/6 -> XVV(6)/1  "<YY(33)>"
  UCVV/1 -> Bus Selector/1
  Bus Selector/1 -> XVV(1)/1  "<YY(28)>"

== system COSTEP/Mixing Zone/Holdup of Components in Mixing Zone/YP(28) ==
  FCM(1,1) : Inport
  FCM(1,2) : Inport  Port=2
  FCM(1,3) : Inport  Port=3
  FCM(1,5) : Inport  Port=4
  FCM(1,9) : Inport  Port=5
  FCM(1,6) : Inport  Port=6
  " " : Sum  Inputs=+++++-
  Bus Selector : BusSelector  OutputSignals=FCM(1;1)
  Bus Selector1 : BusSelector  OutputSignals=FCM(1;2)
  Bus Selector2 : BusSelector  OutputSignals=FCM(1;3)
  Bus Selector3 : BusSelector  OutputSignals=FCM(1;5)
  Bus Selector4 : BusSelector  OutputSignals=FCM(1;9)
  Bus Selector5 : BusSelector  OutputSignals=FCM(1;7)
  Constant : Constant  Value=28
  Initial state variable : mylib/Initial state variable
  Integration : mylib/Integration  SystemSampleTime=-1  VariantActivationTime=update diagram  AllowFlexibleInterface=on  Latency=0  AutoFrameSizeCalculation=off
  YY(28) : Outport  VectorParamsAs1DForOutWhenUnconnected=off
  wires:
  Initial state variable/1 -> Integration/2
  FCM(1,3)/1 -> Bus Selector2/1
  FCM(1,2)/1 -> Bus Selector1/1
  " "/1 -> Integration/1
  Integration/1 -> YY(28)/1
  FCM(1,5)/1 -> Bus Selector3/1
  FCM(1,9)/1 -> Bus Selector4/1
  FCM(1,6)/1 -> Bus Selector5/1
  FCM(1,1)/1 -> Bus Selector/1
  Bus Selector/1 -> " "/1  "<FCM(1;1)>"
  Bus Selector1/1 -> " "/2  "<FCM(1;2)>"
  Bus Selector2/1 -> " "/3  "<FCM(1;3)>"
  Bus Selector3/1 -> " "/4  "<FCM(1;5)>"
  Bus Selector4/1 -> " "/5  "<FCM(1;9)>"
  Bus Selector5/1 -> " "/6  "<FCM(1;7)>"
  Constant/1 -> Initial state variable/1

== system COSTEP/Mixing Zone/Holdup of Components in Mixing Zone/YP(29) ==
  FCM(2,1) : Inport
  FCM(2,2) : Inport  Port=2
  FCM(2,3) : Inport  Port=3
  FCM(2,5) : Inport  Port=4
  FCM(2,9) : Inport  Port=5
  FCM(2,6) : Inport  Port=6
  " " : Sum  Inputs=+++++-
  Bus Selector : BusSelector  OutputSignals=FCM(2;1)
  Bus Selector1 : BusSelector  OutputSignals=FCM(2;2)
  Bus Selector2 : BusSelector  OutputSignals=FCM(2;3)
  Bus Selector3 : BusSelector  OutputSignals=FCM(2;5)
  Bus Selector4 : BusSelector  OutputSignals=FCM(2;9)
  Bus Selector5 : BusSelector  OutputSignals=FCM(2;7)
  Constant : Constant  Value=29
  Initial state variable : mylib/Initial state variable
  Integration : mylib/Integration  SystemSampleTime=-1  VariantActivationTime=update diagram  AllowFlexibleInterface=on  Latency=0  AutoFrameSizeCalculation=off
  YY(29) : Outport  VectorParamsAs1DForOutWhenUnconnected=off
  wires:
  Initial state variable/1 -> Integration/2
  FCM(2,3)/1 -> Bus Selector2/1
  FCM(2,2)/1 -> Bus Selector1/1
  FCM(2,1)/1 -> Bus Selector/1
  " "/1 -> Integration/1
  Integration/1 -> YY(29)/1
  FCM(2,5)/1 -> Bus Selector3/1
  FCM(2,9)/1 -> Bus Selector4/1
  FCM(2,6)/1 -> Bus Selector5/1
  Bus Selector/1 -> " "/1  "<FCM(2;1)>"
  Bus Selector1/1 -> " "/2  "<FCM(2;2)>"
  Bus Selector2/1 -> " "/3  "<FCM(2;3)>"
  Bus Selector3/1 -> " "/4  "<FCM(2;5)>"
  Bus Selector4/1 -> " "/5  "<FCM(2;9)>"
  Bus Selector5/1 -> " "/6  "<FCM(2;7)>"
  Constant/1 -> Initial state variable/1

== system COSTEP/Mixing Zone/Holdup of Components in Mixing Zone/YP(30) ==
  FCM(3,1) : Inport
  FCM(3,2) : Inport  Port=2
  FCM(3,3) : Inport  Port=3
  FCM(3,5) : Inport  Port=4
  FCM(3,9) : Inport  Port=5
  FCM(3,6) : Inport  Port=6
  " " : Sum  Inputs=+++++-
  Bus Selector : BusSelector  OutputSignals=FCM(3;1)
  Bus Selector1 : BusSelector  OutputSignals=FCM(3;2)
  Bus Selector2 : BusSelector  OutputSignals=FCM(3;3)
  Bus Selector3 : BusSelector  OutputSignals=FCM(3;5)
  Bus Selector4 : BusSelector  OutputSignals=FCM(3;9)
  Bus Selector5 : BusSelector  OutputSignals=FCM(3;7)
  Constant : Constant  Value=30
  Initial state variable : mylib/Initial state variable
  Integration : mylib/Integration  SystemSampleTime=-1  VariantActivationTime=update diagram  AllowFlexibleInterface=on  Latency=0  AutoFrameSizeCalculation=off
  YY(30) : Outport  VectorParamsAs1DForOutWhenUnconnected=off
  wires:
  Initial state variable/1 -> Integration/2
  FCM(3,3)/1 -> Bus Selector2/1
  FCM(3,2)/1 -> Bus Selector1/1
  FCM(3,1)/1 -> Bus Selector/1
  " "/1 -> Integration/1
  Integration/1 -> YY(30)/1
  FCM(3,5)/1 -> Bus Selector3/1
  FCM(3,9)/1 -> Bus Selector4/1
  FCM(3,6)/1 -> Bus Selector5/1
  Bus Selector/1 -> " "/1  "<FCM(3;1)>"
  Bus Selector1/1 -> " "/2  "<FCM(3;2)>"
  Bus Selector2/1 -> " "/3  "<FCM(3;3)>"
  Bus Selector3/1 -> " "/4  "<FCM(3;5)>"
  Bus Selector4/1 -> " "/5  "<FCM(3;9)>"
  Bus Selector5/1 -> " "/6  "<FCM(3;7)>"
  Constant/1 -> Initial state variable/1

== system COSTEP/Mixing Zone/Holdup of Components in Mixing Zone/YP(31) ==
  FCM(4,1) : Inport
  FCM(4,2) : Inport  Port=2
  FCM(4,3) : Inport  Port=3
  FCM(4,5) : Inport  Port=4
  FCM(4,9) : Inport  Port=5
  FCM(4,6) : Inport  Port=6
  " " : Sum  Inputs=+++++-
  Bus Selector : BusSelector  OutputSignals=FCM(4;1)
  Bus Selector1 : BusSelector  OutputSignals=FCM(4;2)
  Bus Selector2 : BusSelector  OutputSignals=FCM(4;3)
  Bus Selector3 : BusSelector  OutputSignals=FCM(4;5)
  Bus Selector4 : BusSelector  OutputSignals=FCM(4;9)
  Bus Selector5 : BusSelector  OutputSignals=FCM(4;7)
  Constant : Constant  Value=31
  Initial state variable : mylib/Initial state variable
  Integration : mylib/Integration  SystemSampleTime=-1  VariantActivationTime=update diagram  AllowFlexibleInterface=on  Latency=0  AutoFrameSizeCalculation=off
  YY(31) : Outport  VectorParamsAs1DForOutWhenUnconnected=off
  wires:
  Initial state variable/1 -> Integration/2
  FCM(4,3)/1 -> Bus Selector2/1
  FCM(4,2)/1 -> Bus Selector1/1
  FCM(4,1)/1 -> Bus Selector/1
  " "/1 -> Integration/1
  Integration/1 -> YY(31)/1
  FCM(4,5)/1 -> Bus Selector3/1
  FCM(4,9)/1 -> Bus Selector4/1
  FCM(4,6)/1 -> Bus Selector5/1
  Bus Selector/1 -> " "/1  "<FCM(4;1)>"
  Bus Selector1/1 -> " "/2  "<FCM(4;2)>"
  Bus Selector2/1 -> " "/3  "<FCM(4;3)>"
  Bus Selector3/1 -> " "/4  "<FCM(4;5)>"
  Bus Selector4/1 -> " "/5  "<FCM(4;9)>"
  Bus Selector5/1 -> " "/6  "<FCM(4;7)>"
  Constant/1 -> Initial state variable/1

== system COSTEP/Mixing Zone/Holdup of Components in Mixing Zone/YP(32) ==
  FCM(5,1) : Inport
  FCM(5,2) : Inport  Port=2
  FCM(5,3) : Inport  Port=3
  FCM(5,5) : Inport  Port=4
  FCM(5,9) : Inport  Port=5
  FCM(5,6) : Inport  Port=6
  " " : Sum  Inputs=+++++-
  Bus Selector : BusSelector  OutputSignals=FCM(5;1)
  Bus Selector1 : BusSelector  OutputSignals=FCM(5;2)
  Bus Selector2 : BusSelector  OutputSignals=FCM(5;3)
  Bus Selector3 : BusSelector  OutputSignals=FCM(5;5)
  Bus Selector4 : BusSelector  OutputSignals=FCM(5;9)
  Bus Selector5 : BusSelector  OutputSignals=FCM(5;7)
  Constant : Constant  Value=32
  Initial state variable : mylib/Initial state variable
  Integration : mylib/Integration  SystemSampleTime=-1  VariantActivationTime=update diagram  AllowFlexibleInterface=on  Latency=0  AutoFrameSizeCalculation=off
  YY(32) : Outport  VectorParamsAs1DForOutWhenUnconnected=off
  wires:
  Initial state variable/1 -> Integration/2
  FCM(5,3)/1 -> Bus Selector2/1
  FCM(5,2)/1 -> Bus Selector1/1
  FCM(5,1)/1 -> Bus Selector/1
  " "/1 -> Integration/1
  Integration/1 -> YY(32)/1
  FCM(5,5)/1 -> Bus Selector3/1
  FCM(5,9)/1 -> Bus Selector4/1
  FCM(5,6)/1 -> Bus Selector5/1
  Bus Selector/1 -> " "/1  "<FCM(5;1)>"
  Bus Selector1/1 -> " "/2  "<FCM(5;2)>"
  Bus Selector2/1 -> " "/3  "<FCM(5;3)>"
  Bus Selector3/1 -> " "/4  "<FCM(5;5)>"
  Bus Selector4/1 -> " "/5  "<FCM(5;9)>"
  Bus Selector5/1 -> " "/6  "<FCM(5;7)>"
  Constant/1 -> Initial state variable/1

== system COSTEP/Mixing Zone/Holdup of Components in Mixing Zone/YP(33) ==
  FCM(6,1) : Inport
  FCM(6,2) : Inport  Port=2
  FCM(6,3) : Inport  Port=3
  FCM(6,5) : Inport  Port=4
  FCM(6,9) : Inport  Port=5
  FCM(6,6) : Inport  Port=6
  " " : Sum  Inputs=+++++-
  Bus Selector : BusSelector  OutputSignals=FCM(6;1)
  Bus Selector1 : BusSelector  OutputSignals=FCM(6;2)
  Bus Selector2 : BusSelector  OutputSignals=FCM(6;3)
  Bus Selector3 : BusSelector  OutputSignals=FCM(6;5)
  Bus Selector4 : BusSelector  OutputSignals=FCM(6;9)
  Bus Selector5 : BusSelector  OutputSignals=FCM(6;7)
  Constant : Constant  Value=33
  Initial state variable : mylib/Initial state variable
  Integration : mylib/Integration  SystemSampleTime=-1  VariantActivationTime=update diagram  AllowFlexibleInterface=on  Latency=0  AutoFrameSizeCalculation=off
  YY(33) : Outport  VectorParamsAs1DForOutWhenUnconnected=off
  wires:
  Initial state variable/1 -> Integration/2
  FCM(6,3)/1 -> Bus Selector2/1
  FCM(6,2)/1 -> Bus Selector1/1
  FCM(6,1)/1 -> Bus Selector/1
  " "/1 -> Integration/1
  Integration/1 -> YY(33)/1
  FCM(6,5)/1 -> Bus Selector3/1
  FCM(6,9)/1 -> Bus Selector4/1
  FCM(6,6)/1 -> Bus Selector5/1
  Bus Selector/1 -> " "/1  "<FCM(6;1)>"
  Bus Selector1/1 -> " "/2  "<FCM(6;2)>"
  Bus Selector2/1 -> " "/3  "<FCM(6;3)>"
  Bus Selector3/1 -> " "/4  "<FCM(6;5)>"
  Bus Selector4/1 -> " "/5  "<FCM(6;9)>"
  Bus Selector5/1 -> " "/6  "<FCM(6;7)>"
  Constant/1 -> Initial state variable/1

== system COSTEP/Mixing Zone/Holdup of Components in Mixing Zone/YP(34) ==
  FCM(7,1) : Inport
  FCM(7,2) : Inport  Port=2
  FCM(7,3) : Inport  Port=3
  FCM(7,5) : Inport  Port=4
  FCM(7,9) : Inport  Port=5
  FCM(7,6) : Inport  Port=6
  " " : Sum  Inputs=+++++-
  Bus Selector : BusSelector  OutputSignals=FCM(7;1)
  Bus Selector1 : BusSelector  OutputSignals=FCM(7;2)
  Bus Selector2 : BusSelector  OutputSignals=FCM(7;3)
  Bus Selector3 : BusSelector  OutputSignals=FCM(7;5)
  Bus Selector4 : BusSelector  OutputSignals=FCM(7;9)
  Bus Selector5 : BusSelector  OutputSignals=FCM(7;7)
  Constant : Constant  Value=34
  Initial state variable : mylib/Initial state variable
  Integration : mylib/Integration  SystemSampleTime=-1  VariantActivationTime=update diagram  AllowFlexibleInterface=on  Latency=0  AutoFrameSizeCalculation=off
  YY(34) : Outport  VectorParamsAs1DForOutWhenUnconnected=off
  wires:
  Initial state variable/1 -> Integration/2
  FCM(7,3)/1 -> Bus Selector2/1
  FCM(7,2)/1 -> Bus Selector1/1
  FCM(7,1)/1 -> Bus Selector/1
  " "/1 -> Integration/1
  Integration/1 -> YY(34)/1
  FCM(7,5)/1 -> Bus Selector3/1
  FCM(7,9)/1 -> Bus Selector4/1
  FCM(7,6)/1 -> Bus Selector5/1
  Bus Selector/1 -> " "/1  "<FCM(7;1)>"
  Bus Selector1/1 -> " "/2  "<FCM(7;2)>"
  Bus Selector2/1 -> " "/3  "<FCM(7;3)>"
  Bus Selector3/1 -> " "/4  "<FCM(7;5)>"
  Bus Selector4/1 -> " "/5  "<FCM(7;9)>"
  Bus Selector5/1 -> " "/6  "<FCM(7;7)>"
  Constant/1 -> Initial state variable/1

== system COSTEP/Mixing Zone/Holdup of Components in Mixing Zone/YP(35) ==
  FCM(8,1) : Inport
  FCM(8,2) : Inport  Port=2
  FCM(8,3) : Inport  Port=3
  FCM(8,5) : Inport  Port=4
  FCM(8,9) : Inport  Port=5
  FCM(8,6) : Inport  Port=6
  " " : Sum  Inputs=+++++-
  Bus Selector : BusSelector  OutputSignals=FCM(8;1)
  Bus Selector1 : BusSelector  OutputSignals=FCM(8;2)
  Bus Selector2 : BusSelector  OutputSignals=FCM(8;3)
  Bus Selector3 : BusSelector  OutputSignals=FCM(8;5)
  Bus Selector4 : BusSelector  OutputSignals=FCM(8;9)
  Bus Selector5 : BusSelector  OutputSignals=FCM(8;7)
  Constant : Constant  Value=35
  Initial state variable : mylib/Initial state variable
  Integration : mylib/Integration  SystemSampleTime=-1  VariantActivationTime=update diagram  AllowFlexibleInterface=on  Latency=0  AutoFrameSizeCalculation=off
  YY(35) : Outport  VectorParamsAs1DForOutWhenUnconnected=off
  wires:
  Initial state variable/1 -> Integration/2
  FCM(8,3)/1 -> Bus Selector2/1
  FCM(8,2)/1 -> Bus Selector1/1
  FCM(8,1)/1 -> Bus Selector/1
  " "/1 -> Integration/1
  Integration/1 -> YY(35)/1
  FCM(8,5)/1 -> Bus Selector3/1
  FCM(8,9)/1 -> Bus Selector4/1
  FCM(8,6)/1 -> Bus Selector5/1
  Bus Selector/1 -> " "/1  "<FCM(8;1)>"
  Bus Selector1/1 -> " "/2  "<FCM(8;2)>"
  Bus Selector2/1 -> " "/3  "<FCM(8;3)>"
  Bus Selector3/1 -> " "/4  "<FCM(8;5)>"
  Bus Selector4/1 -> " "/5  "<FCM(8;9)>"
  Bus Selector5/1 -> " "/6  "<FCM(8;7)>"
  Constant/1 -> Initial state variable/1

== system COSTEP/Mixing Zone/Stream 6/HST(6) Molar Enthalpy of Stream 6 MBtu//lb-mol ==
  ITY : Inport
  T : Inport  Port=2
  XST(I,6) : Inport  Port=3
  "Enthalpy of Stream " : mylib/Enthalpy of Stream   SystemSampleTime=-1  VariantActivationTime=update diagram  AllowFlexibleInterface=on  Latency=0  AutoFrameSizeCalculation=off
  "H " : Outport  VectorParamsAs1DForOutWhenUnconnected=off
  wires:
  ITY/1 -> "Enthalpy of Stream "/1
  T/1 -> "Enthalpy of Stream "/2
  XST(I,6)/1 -> "Enthalpy of Stream "/3
  "Enthalpy of Stream "/1 -> "H "/1

== system COSTEP/Mixing Zone/Stream 6/Subsystem ==
  Abs : Abs  SaturateOnIntegerOverflow=off
  Constant : Constant  Value=0.0
  Constant1 : Constant  Value=1937.6
  DLP : Sum  Inputs=+-
  DLP Pressure drop between reactor and mixing zone : Merge
  FLMS : Product
  If : If  IfExpression=u1 < 0
  If Action Subsystem : Subsystem  TreatAsAtomicUnit=on
  If Action Subsystem1 : Subsystem  TreatAsAtomicUnit=on
  Sqrt : Sqrt
  "FLMS " : Outport  VectorParamsAs1DForOutWhenUnconnected=off
  wires:
  [PTR] -> DLP/2
  Abs/1 -> Sqrt/1
  Constant1/1 -> FLMS/1
  If Action Subsystem/1(Out1) -> DLP Pressure drop between reactor and mixing zone/1
  If Action Subsystem1/1(Out1) -> DLP Pressure drop between reactor and mixing zone/2
  [PTV] -> DLP/1
  Constant/1 -> If Action Subsystem/1(In1)
  Sqrt/1 -> FLMS/2
  DLP/1 -> If Action Subsystem1/1(In1), If/1
  If/1 -> If Action Subsystem/Action
  DLP Pressure drop between reactor and mixing zone/1 -> Abs/1
  If/2 -> If Action Subsystem1/Action
  FLMS/1 -> "FLMS "/1

== system COSTEP/Mixing Zone/Stream 6/XMWS(6) Molecular weight of Stream 6 lb//lb-mol ==
  XST(I,6) : Inport
  Product : Product
  Sum of Elements : Sum  Inputs=+
  "XMW(I) Molecular weight of components lb/lb-mol " : Constant  Value=XMW
  XMWS(6) : Outport  VectorParamsAs1DForOutWhenUnconnected=off
  wires:
  Sum of Elements/1 -> XMWS(6)/1
  Product/1 -> Sum of Elements/1
  XST(I,6)/1 -> Product/1
  "XMW(I) Molecular weight of components lb/lb-mol "/1 -> Product/2

== system COSTEP/Process Measurements/Feed Streams/ A Feed ==
  " " : Constant  Value=35.3145
  "  " : Constant  Value=0.359
  Add : Sum
  Bus Selector : BusSelector  OutputSignals=FTM(3)
  Bus Selector1 : BusSelector  OutputSignals=XMNS(1)
  Product1 : Product  Inputs=**/
  "XMEAS(1) " : Outport  PortDimensions=1  VectorParamsAs1DForOutWhenUnconnected=off
  wires:
  " "/1 -> Product1/3
  "  "/1 -> Product1/2
  [PropertiesStream3] -> Bus Selector/1
  Bus Selector/1 -> Product1/1  "<FTM(3)>"
  Product1/1 -> Add/1
  Add/1 -> "XMEAS(1) "/1  "XMEAS(1)"
  [XMNS] -> Bus Selector1/1
  Bus Selector1/1 -> Add/2  "<XMNS(1)>"

== system COSTEP/Process Measurements/Feed Streams/A and C Feed ==
  " " : Constant  Value=35.3145
  "  " : Constant  Value=0.359
  Add : Sum
  Bus Selector : BusSelector  OutputSignals=FTM(4)
  Bus Selector1 : BusSelector  OutputSignals=XMNS(4)
  Product1 : Product  Inputs=**/
  "XMEAS(4) " : Outport  PortDimensions=1  VectorParamsAs1DForOutWhenUnconnected=off
  wires:
  " "/1 -> Product1/3
  "  "/1 -> Product1/2
  [PropertiesStream4] -> Bus Selector/1
  Bus Selector/1 -> Product1/1  "<FTM(4)>"
  Bus Selector1/1 -> Add/2  "<XMNS(4)>"
  Product1/1 -> Add/1
  Add/1 -> "XMEAS(4) "/1  "XMEAS(4)"
  [XMNS] -> Bus Selector1/1

== system COSTEP/Process Measurements/Feed Streams/D Feed ==
  Add : Sum
  Bus Selector : BusSelector  OutputSignals=XST(I;1),FTM(1)
  Bus Selector1 : BusSelector  OutputSignals=XMNS(2)
  Convert from lb/h to kg/h : Constant  Value=0.454
  Product : Product  Inputs=3
  XMWS(1) Molecular weight of Stream 1 lb/lb-mol : Subsystem
  "XMEAS(2) " : Outport  VectorParamsAs1DForOutWhenUnconnected=off
  wires:
  Convert from lb/h to kg/h/1 -> Product/3
  XMWS(1) Molecular weight of Stream 1 lb/lb-mol/1(XMWS(1)) -> Product/1
  [PropertiesStream1] -> Bus Selector/1
  Bus Selector/2 -> Product/2  "<FTM(1)>"
  Bus Selector/1 -> XMWS(1) Molecular weight of Stream 1 lb/lb-mol/1(XST(I,1))  "<XST(I;1)>"
  Bus Selector1/1 -> Add/2  "<XMNS(2)>"
  Product/1 -> Add/1
  Add/1 -> "XMEAS(2) "/1  "XMEAS(2)"
  [XMNS] -> Bus Selector1/1

== system COSTEP/Process Measurements/Feed Streams/E Feed ==
  Add : Sum
  Bus Selector : BusSelector  OutputSignals=XST(I;2),FTM(2)
  Bus Selector1 : BusSelector  OutputSignals=XMNS(3)
  Convert from lb/h to kg/h : Constant  Value=0.454
  Product : Product  Inputs=3
  XMWS(2) Molecular weight of Stream 2 lb/lb-mol : Subsystem
  "XMEAS(3) " : Outport  VectorParamsAs1DForOutWhenUnconnected=off
  wires:
  Convert from lb/h to kg/h/1 -> Product/3
  Bus Selector/1 -> XMWS(2) Molecular weight of Stream 2 lb/lb-mol/1(XST(I,2))  "<XST(I;2)>"
  XMWS(2) Molecular weight of Stream 2 lb/lb-mol/1(XMWS(2)) -> Product/1
  Bus Selector/2 -> Product/2  "<FTM(2)>"
  [PropertiesStream2] -> Bus Selector/1
  Bus Selector1/1 -> Add/2  "<XMNS(3)>"
  Product/1 -> Add/1
  Add/1 -> "XMEAS(3) "/1  "XMEAS(3)"
  [XMNS] -> Bus Selector1/1

== system COSTEP/Process Measurements/Feed Streams/Recycle Flow ==
  " " : Constant  Value=35.3145
  "  " : Constant  Value=0.359
  Add : Sum
  Bus Selector : BusSelector  OutputSignals=signal2.FTM(9)
  Bus Selector1 : BusSelector  OutputSignals=XMNS(5)
  Product1 : Product  Inputs=**/
  "XMEAS(5) " : Outport  VectorParamsAs1DForOutWhenUnconnected=off
  wires:
  " "/1 -> Product1/3
  Bus Selector/1 -> Product1/1  "<FTM(9)>"
  "  "/1 -> Product1/2
  [PropertiesStream9] -> Bus Selector/1
  Bus Selector1/1 -> Add/2  "<XMNS(5)>"
  Product1/1 -> Add/1
  Add/1 -> "XMEAS(5) "/1  "XMEAS(5)"
  [XMNS] -> Bus Selector1/1
